simulink model "testingexciter"  (R2016b)
settings: Solver=ode1  StartTime=0.0  StopTime=10.0  FixedStep=1e-3  RelTol=1e-3
values from neighbouring files (symbols this model uses):
  Te = csvread('../../vsa/Results/SynGenVBREmt_ABCFault_DPsim_1_Damping/data_synGenVBR_Te.csv')    [compareDPresults_with_PLECS.m]
undefined symbols (not defined in the file or in its folder): Ka, Ke, Kf, Ta, Tf, Tr
settings Model: Creator=mmi-vsa  LastModifiedBy=mmi-vsa

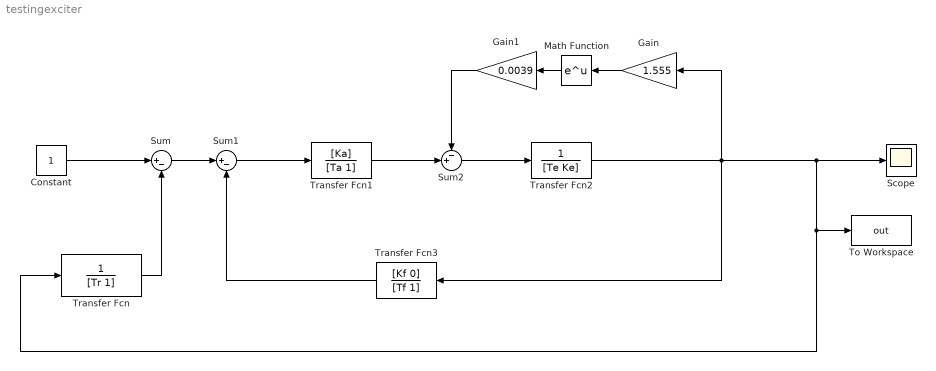
== system testingexciter ==
  Constant : Constant
  Gain : Gain  Gain=1.555
  Gain1 : Gain  Gain=0.0039
  Math Function : Math  SaturateOnIntegerOverflow=on
  Scope : Scope
  Sum : Sum  Inputs=|+-
  Sum1 : Sum  Inputs=|+-
  Sum2 : Sum  Inputs=-+|
  To Workspace : ToWorkspace  VariableName=out  SampleTime=-1
  Transfer Fcn : TransferFcn  Denominator=[Tr 1]
  Transfer Fcn1 : TransferFcn  Numerator=[Ka]  Denominator=[Ta 1]
  Transfer Fcn2 : TransferFcn  Denominator=[Te Ke]
  Transfer Fcn3 : TransferFcn  Numerator=[Kf 0]  Denominator=[Tf 1]
  wires:
  Transfer Fcn/1 -> Sum/2
  Sum/1 -> Sum1/1
  Sum1/1 -> Transfer Fcn1/1
  Sum2/1 -> Transfer Fcn2/1
  Transfer Fcn1/1 -> Sum2/2
  Math Function/1 -> Gain1/1
  Transfer Fcn3/1 -> Sum1/2
  Constant/1 -> Sum/1
  Gain1/1 -> Sum2/1
  Gain/1 -> Math Function/1
  Transfer Fcn2/1 -> To Workspace/1, Transfer Fcn/1, Scope/1, Transfer Fcn3/1, Gain/1
